simulink model "Serial_sm"  (R2021a)
settings: Solver=ode4  StartTime=0.0  StopTime=inf  FixedStep=0.01  RelTol=1e-3
undefined symbols (not defined in the file): LF
libraries: instrumentseriallib x2
settings Model: Creator=josed  LastModifiedBy=josed

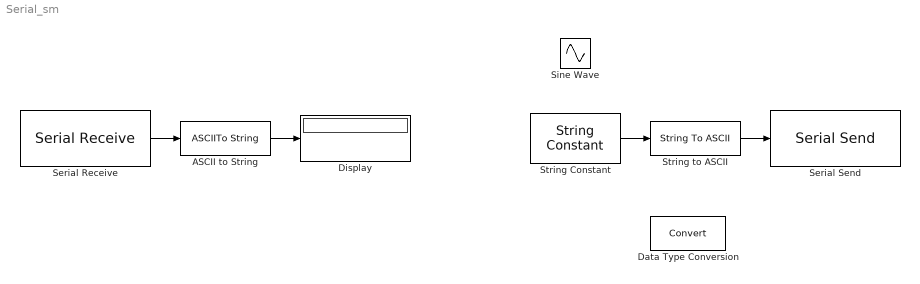
== system Serial_sm ==
  ASCII to String : ASCIIToString
  Data Type Conversion : DataTypeConversion
  Display : Display
  Serial Receive : instrumentseriallib/Serial Receive  Priority=1  Port=<Select a port...>  ComPort=<Select a port...>  DataType=uint8  SaveDataType=uint8  ToggleHeader=off  Header='A'  ToggleTerminator=on  Terminator=LF ('\n')  CustomTerminator=[]  ToggleDataSize=on  DataSize=[1 1]  EnableBlockingMode=on  ActionDataUnavailable=Output custom value  ActionWhenDataUnavailable=Output custom value  CustomValue=9  SampleTime=0.05  SimulateUsing=Interpreted execution  BlockInModel=on
  Serial Send : instrumentseriallib/Serial Send  Priority=1  Port=<Select a port...>  ComPort=<Select a port...>  Header=[]  Terminator=LF ('\n')  CustomTerminator=[]  EnableBlockingMode=on  SimulateUsing=Interpreted execution  BlockInModel=on
  Sine Wave : Sin  SampleTime=0
  String Constant : StringConstant
  String to ASCII : StringToASCII
  wires:
  String Constant/1 -> String to ASCII/1
  ASCII to String/1 -> Display/1
  Serial Receive/1 -> ASCII to String/1
  String to ASCII/1 -> Serial Send/1
